simulink library "ss_angles_2_vec"  (R2018b)
settings: Solver=VariableStepAuto  StartTime=0.0  StopTime=10.0  RelTol=1e-3
undefined symbols (not defined in the file or in its folder): simParams
libraries: simulink x2
settings Model: Creator=taylorreynolds  LastModifiedBy=Taylor
settings SFSimCC: SimUseLocalCustomCode=off
settings RTWCC: RTWUseLocalCustomCode=off
settings CodeAppCC: StateflowObjectComments=on

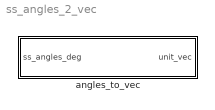
== system ss_angles_2_vec ==
  angles_to_vec : Subsystem

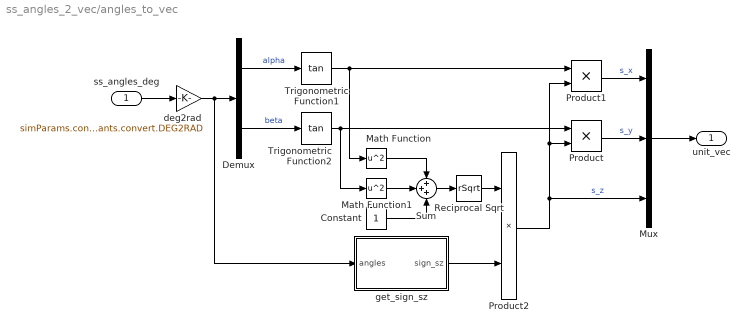
== system ss_angles_2_vec/angles_to_vec ==
  ss_angles_deg : Inport
  Constant : Constant
  Demux : Demux  Outputs=[1 1]
  Math Function : Math  Operator=square  SaturateOnIntegerOverflow=on
  Math Function1 : Math  Operator=square  SaturateOnIntegerOverflow=on
  Mux : Mux  Inputs=3
  Product : Product
  Product1 : Product
  Product2 : Product
  Reciprocal Sqrt : Sqrt  Operator=rSqrt  SaturateOnIntegerOverflow=on
  Sum : Sum  Inputs=+++
  Trigonometric Function1 : Trigonometry  Operator=tan  OutputSignalType=real
  Trigonometric Function2 : Trigonometry  Operator=tan  OutputSignalType=real
  deg2rad : Gain  Gain=simParams.constants.convert.DEG2RAD
  get_sign_sz : Subsystem
  unit_vec : Outport
  wires:
  get_sign_sz/1(sign_sz) -> Product2/2
  Reciprocal Sqrt/1 -> Product2/1
  Product2/1 -> Mux/3, Product/2, Product1/2  "s_z"
  ss_angles_deg/1 -> deg2rad/1
  Product1/1 -> Mux/1  "s_x"
  Product/1 -> Mux/2  "s_y"
  Mux/1 -> unit_vec/1
  deg2rad/1 -> Demux/1, get_sign_sz/1(angles)
  Demux/1 -> Trigonometric Function1/1  "alpha"
  Sum/1 -> Reciprocal Sqrt/1
  Constant/1 -> Sum/3
  Math Function1/1 -> Sum/2
  Math Function/1 -> Sum/1
  Demux/2 -> Trigonometric Function2/1  "beta"
  Trigonometric Function1/1 -> Product1/1, Math Function/1
  Trigonometric Function2/1 -> Product/1, Math Function1/1

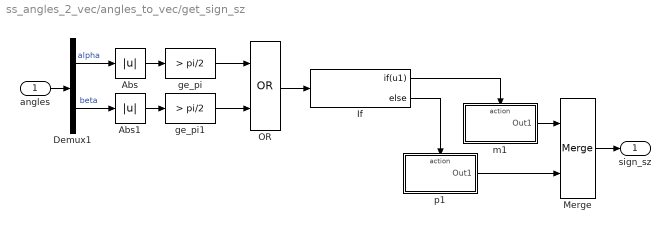
== system ss_angles_2_vec/angles_to_vec/get_sign_sz ==
  angles : Inport
  Abs : Abs
  Abs1 : Abs
  Demux1 : Demux  Outputs=[1 1]
  If : If  IfExpression=u1
  Merge : Merge
  OR : Logic  Operator=OR  AllPortsSameDT=off  OutDataTypeStr=boolean
  ge_pi : simulink/Logic and Bit Operations/Compare To Constant  relop=>  const=pi/2  OutDataTypeStr=boolean
  ge_pi1 : simulink/Logic and Bit Operations/Compare To Constant  relop=>  const=pi/2  OutDataTypeStr=boolean
  m1 : Subsystem  TreatAsAtomicUnit=on
  p1 : Subsystem  TreatAsAtomicUnit=on
  sign_sz : Outport
  wires:
  Abs1/1 -> ge_pi1/1
  Abs/1 -> ge_pi/1
  Merge/1 -> sign_sz/1
  p1/1(Out1) -> Merge/2
  m1/1(Out1) -> Merge/1
  If/2 -> p1/Action
  If/1 -> m1/Action
  OR/1 -> If/1
  Demux1/1 -> Abs/1  "alpha"
  Demux1/2 -> Abs1/1  "beta"
  angles/1 -> Demux1/1
  ge_pi/1 -> OR/1
  ge_pi1/1 -> OR/2

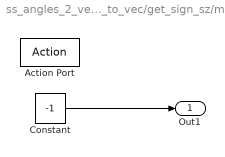
== system ss_angles_2_vec/angles_to_vec/get_sign_sz/m1 ==
  Action Port : ActionPort
  Constant : Constant  Value=-1
  Out1 : Outport
  wires:
  Constant/1 -> Out1/1

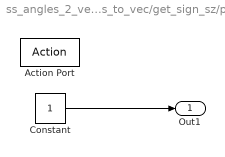
== system ss_angles_2_vec/angles_to_vec/get_sign_sz/p1 ==
  Action Port : ActionPort
  Constant : Constant
  Out1 : Outport
  wires:
  Constant/1 -> Out1/1
